simulink model "pendulum1"  (R2014a)
settings: Solver=ode45  StartTime=0.0  StopTime=simTime  MaxStep=0.001  RelTol=1e-3
settings Model: Creator=Ash  LastModifiedBy=Ash
settings DataIOCC: ExternalInput=Input  LimitDataPoints=off  LoadExternalInput=on  OutputSaveName=r, r_d, s, s_d, r_dd, s_dd, x_dd_out, y_dd_out, z_dd_out

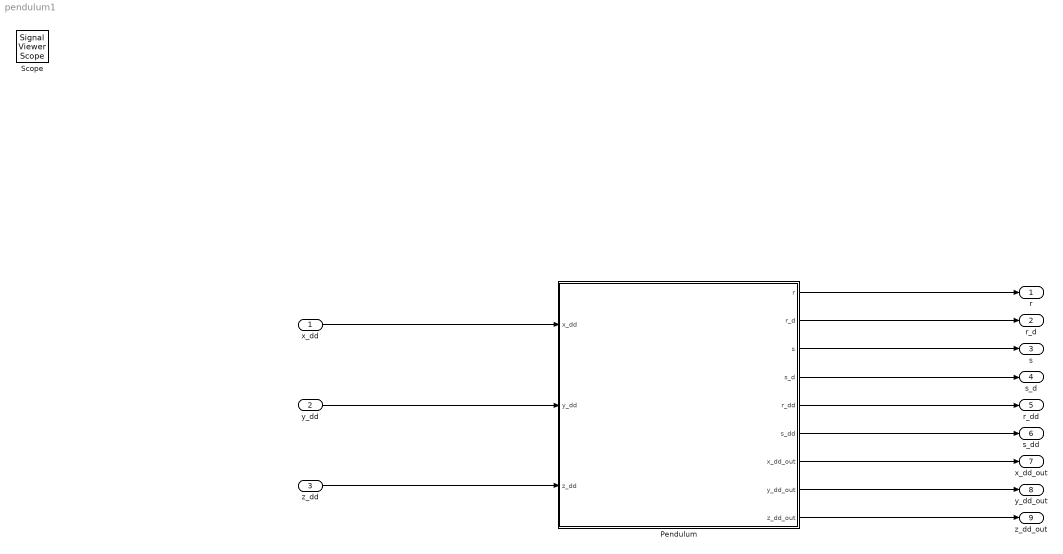
== system pendulum1 ==
  x_dd : Inport
  y_dd : Inport  Port=2
  z_dd : Inport  Port=3
  Pendulum : Subsystem
  r : Outport
  r_d : Outport  Port=2
  s : Outport  Port=3
  s_d : Outport  Port=4
  r_dd : Outport  Port=5
  s_dd : Outport  Port=6
  x_dd_out : Outport  Port=7
  y_dd_out : Outport  Port=8
  z_dd_out : Outport  Port=9
  Scope : SignalViewerScope  IOType=viewer  LegendLocations="0.96635     0.93568    0.028125    0.041641"  RefreshTime=0.035000
      settings: ShowLegends=on
  wires:
  x_dd/1 -> Pendulum/1(x_dd)
  y_dd/1 -> Pendulum/2(y_dd)
  z_dd/1 -> Pendulum/3(z_dd)
  Pendulum/1(r) -> r/1
  Pendulum/2(r_d) -> r_d/1
  Pendulum/4(s_d) -> s_d/1
  Pendulum/3(s) -> s/1
  Pendulum/5(r_dd) -> r_dd/1
  Pendulum/6(s_dd) -> s_dd/1
  Pendulum/7(x_dd_out) -> x_dd_out/1
  Pendulum/8(y_dd_out) -> y_dd_out/1
  Pendulum/9(z_dd_out) -> z_dd_out/1

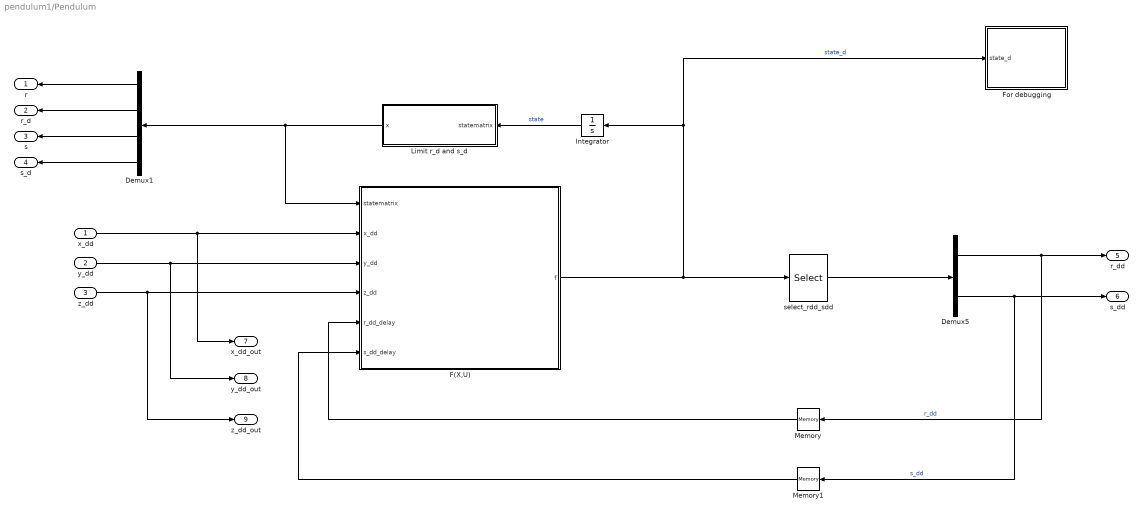
== system pendulum1/Pendulum ==
  x_dd : Inport
  y_dd : Inport  Port=2
  z_dd : Inport  Port=3
  Demux1 : Demux  Outputs=[1 1 1 1]
  Demux5 : Demux  Outputs=[1 1]
  F(X,U) : MATLAB Function  TreatAsAtomicUnit=on
  For debugging : Subsystem
  Integrator : Integrator
  Limit r_d and s_d : MATLAB Function  TreatAsAtomicUnit=on
  Memory : Memory
  Memory1 : Memory
  select_rdd_sdd : Selector  InputPortWidth=4  Indices=[2 4]
  r : Outport
  r_d : Outport  Port=2
  s : Outport  Port=3
  s_d : Outport  Port=4
  r_dd : Outport  Port=5
  s_dd : Outport  Port=6
  x_dd_out : Outport  Port=7
  y_dd_out : Outport  Port=8
  z_dd_out : Outport  Port=9
  wires:
  Memory1/1 -> F(X,U)/6(s_dd_delay)
  Demux5/1 -> r_dd/1, Memory/1  "r_dd"
  Memory/1 -> F(X,U)/5(r_dd_delay)
  select_rdd_sdd/1 -> Demux5/1
  Demux5/2 -> s_dd/1, Memory1/1  "s_dd"
  z_dd/1 -> F(X,U)/4(z_dd), z_dd_out/1
  y_dd/1 -> F(X,U)/3(y_dd), y_dd_out/1
  Demux1/1 -> r/1
  Demux1/2 -> r_d/1
  Demux1/4 -> s_d/1
  Demux1/3 -> s/1
  F(X,U)/1(f) -> For debugging/1(state_d), Integrator/1, select_rdd_sdd/1  "state_d"
  x_dd/1 -> F(X,U)/2(x_dd), x_dd_out/1
  Limit r_d and s_d/1(x) -> F(X,U)/1(statematrix), Demux1/1
  Integrator/1 -> Limit r_d and s_d/1(statematrix)  "state"

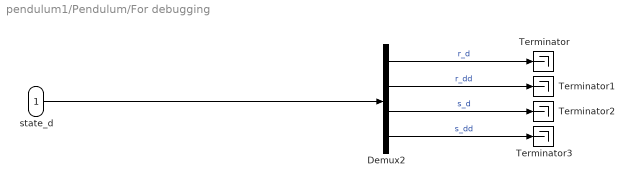
== system pendulum1/Pendulum/For debugging ==
  state_d : Inport
  Demux2 : Demux  Outputs=[1 1 1 1]
  Terminator{,1..3} (4 alike) : Terminator
  wires:
  Demux2/4 -> Terminator3/1  "s_dd"
  Demux2/3 -> Terminator2/1  "s_d"
  Demux2/2 -> Terminator1/1  "r_dd"
  Demux2/1 -> Terminator/1  "r_d"
  state_d/1 -> Demux2/1

== matlab function pendulum1/Pendulum/Limit r_d and s_d ==
  data: statematrix input; x output
function x = fcn(statematrix)

L = 0.4;

r = statematrix(1);
r_d = statematrix(2);
s = statematrix (3);
s_d = statematrix(4);

if ((r^2 + s^2) > (L^2))
    
    r_d = 0;
    s_d = 0;
    
end

x = [r; r_d; s; s_d];

== matlab function pendulum1/Pendulum/F(X,U) ==
  data: statematrix input; x_dd input; y_dd input; z_dd input; r_dd_delay input; s_dd_delay input; f output
function f = fcn(statematrix, x_dd, y_dd, z_dd, r_dd_delay, s_dd_delay)

g = -9.81;
L = 0.4;

r = statematrix(1);
r_d = statematrix(2);
s = statematrix(3);
s_d = statematrix(4);

if ((r^2 + s^2) <= (L^2))
    
    zeta = sqrt(L^2 - r^2 - s^2);
    r_dd = (1/((L^2 - s^2)*zeta)) * ( -r^4*x_dd - (L^2 - s^2)^2*x_dd - 2*r^2*(s*r_d*s_d + (-L^2 + s^2)*x_dd) + r^3*(s_d^2 + s*s_dd_delay - zeta*(g+z_dd)) + r*(-L^2*s*s_dd_delay + s^3*s_dd_delay + s^2*(r_d^2 - zeta*(g+z_dd)) + L^2*(-r_d^2 - s_d^2 + zeta*(g+z_dd))) );
    s_dd = (1/((L^2 - r^2)*zeta)) * ( -s^4*y_dd - (L^2 - r^2)^2*y_dd - 2*s^2*(r*r_d*s_d + (-L^2 + r^2)*y_dd) + s^3*(r_d^2 + r*r_dd_delay - zeta*(g+z_dd)) + s*(-L^2*r*r_dd_delay + r^3*r_dd_delay + r^2*(s_d^2 - zeta*(g+z_dd)) + L^2*(-r_d^2 - s_d^2 + zeta*(g+z_dd))) );

    
else
    
    r_d = 0;
    s_d = 0;
    r_dd = 0;
    s_dd = 0;
    
end


f = [r_d; r_dd; s_d; s_dd];
